simulink model "OL_HiLData"  (R2015b)
settings: Solver=FixedStepDiscrete  StartTime=0.0  StopTime=stop_time  FixedStep=step_size  RelTol=1e-3
values from neighbouring files (symbols this model uses):
  step_size = 0.1    [loadCalib.m]
  stop_time = 660    [run_test_cases.m]
undefined symbols (not defined in the file or in its folder): canChannel
libraries: canmsglib x62, canlib x29, realtime_pacer_lib x1
(part 2 of 4)

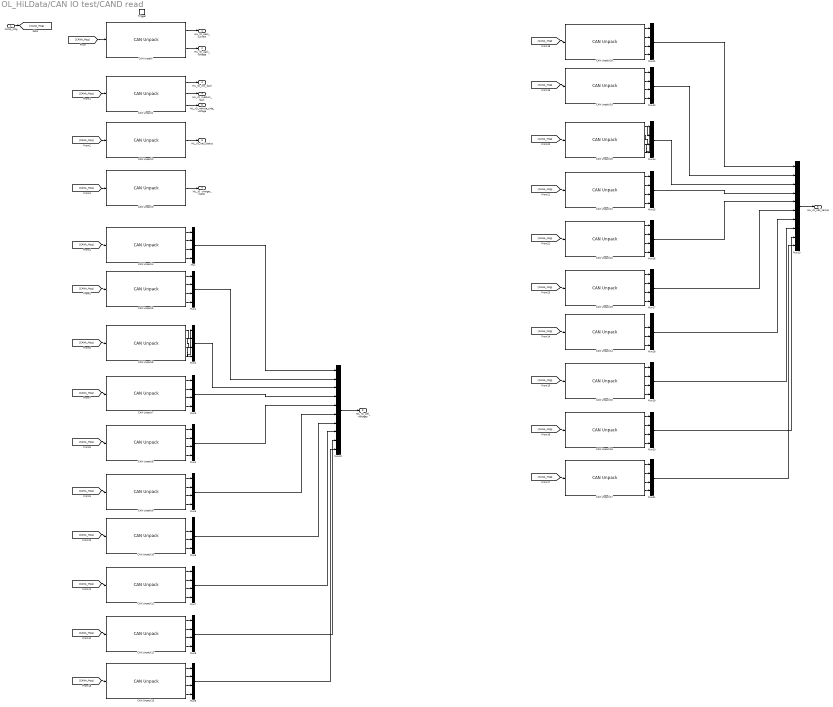
== system OL_HiLData/CAN IO test/CAND read ==
  CANA_Msg : Inport
  Trigger : TriggerPort  TriggerType=function-call  PortDimensions=1
  CAN Unpack : canmsglib/CAN Unpack  CANdbFile=D:\Projects\BMS\P006n\08_Work_in_progress\Repo_Sync_folder\HiLCANIO\IOdb.dbc  MsgList=pack_data  MsgName=pack_data  MsgIDType=Standard (11-bit identifier)  MsgIdentifier=113  MsgLength=8  SignalInfo=pack_current$16$24$2$1$1$0$1.000000e-03$0$-200$200$#pack_voltage$40$24$2$2$1$0$1.000000e-03$0$0$200$#  NSignals=2  IDPort=off  TimestampPort=off  ErrorPort=off  RemotePort=off  LengthPort=off  StatusPort=off  StartBits=str2num('[int32(16);int32(40)]')  SignalSizes=str2num('[int32(24);int32(24)]')  ByteOrders=str2num('[int32(2);int32(2)]')  DataTypes=str2num('[int32(1);int32(2)]')  MultiplexTypes=str2num('[int32(1);int32(1)]')  MultiplexValues=str2num('[double(0);double(0)]')  Factors=str2num('[double(1.000000e-03);double(1.000000e-03)]')  Offsets=str2num('[double(0);double(0)]')  Minimums=str2num('[double(-200);double(0)]')  Maximums=str2num('[double(200);double(200)]')
      settings: DataFormat=CANdb specified signals
  CAN Unpack1 : canmsglib/CAN Unpack  CANdbFile=D:\Projects\BMS\P006n\08_Work_in_progress\Repo_Sync_folder\HiLCANIO\IOdb.dbc  MsgList=pack_data_2  MsgName=pack_data_2  MsgIDType=Standard (11-bit identifier)  MsgIdentifier=114  MsgLength=8  SignalInfo=low_fault$30$1$2$2$1$0$1$0$0$1$#medium_fault$31$1$2$2$1$0$1$0$0$1$#vehicle_side_voltage$16$24$2$2$1$0$1$0$0$200$#  NSignals=3  IDPort=off  TimestampPort=off  ErrorPort=off  RemotePort=off  LengthPort=off  StatusPort=off  StartBits=str2num('[int32(30);int32(31);int32(16)]')  SignalSizes=str2num('[int32(1);int32(1);int32(24)]')  ByteOrders=str2num('[int32(2);int32(2);int32(2)]')  DataTypes=str2num('[int32(2);int32(2);int32(2)]')  MultiplexTypes=str2num('[int32(1);int32(1);int32(1)]')  MultiplexValues=str2num('[double(0);double(0);double(0)]')  Factors=str2num('[double(1);double(1);double(1)]')  Offsets=str2num('[double(0);double(0);double(0)]')  Minimums=str2num('[double(0);double(0);double(0)]')  Maximums=str2num('[double(1);double(1);double(200)]')
      settings: DataFormat=CANdb specified signals
  CAN Unpack10 : canmsglib/CAN Unpack  CANdbFile=D:\Projects\BMS\P006n\08_Work_in_progress\Repo_Sync_folder\HiLCANIO\IOdb.dbc  MsgList=cell_voltage_25_28  MsgName=cell_voltage_25_28  MsgIDType=Standard (11-bit identifier)  MsgIdentifier=86  MsgLength=8  SignalInfo=cell25_votlage$8$16$2$2$1$0$1.000000e-04$0$0$5$#cell26_votlage$24$16$2$2$1$0$1.000000e-04$0$0$5$#cell27_votlage$40$16$2$2$1$0$1.000000e-04$0$0$5$#cell28_votlage$56$16$2$2$1$0$1.000000e-04$0$0$5$#  NSignals=4  IDPort=off  TimestampPort=off  ErrorPort=off  RemotePort=off  LengthPort=off  StatusPort=off  StartBits=str2num('[int32(8);int32(24);int32(40);int32(56)]')  SignalSizes=str2num('[int32(16);int32(16);int32(16);int32(16)]')  ByteOrders=str2num('[int32(2);int32(2);int32(2);int32(2)]')  DataTypes=str2num('[int32(2);int32(2);int32(2);int32(2)]')  MultiplexTypes=str2num('[int32(1);int32(1);int32(1);int32(1)]')  MultiplexValues=str2num('[double(0);double(0);double(0);double(0)]')  Factors=str2num('[double(1.000000e-04);double(1.000000e-04);double(1.000000e-04);double(1.000000e-04)]')  Offsets=str2num('[double(0);double(0);double(0);double(0)]')  Minimums=str2num('[double(0);double(0);double(0);double(0)]')  Maximums=str2num('[double(5);double(5);double(5);double(5)]')
      settings: DataFormat=CANdb specified signals
  CAN Unpack11 : canmsglib/CAN Unpack  CANdbFile=D:\Projects\BMS\P006n\08_Work_in_progress\Repo_Sync_folder\HiLCANIO\IOdb.dbc  MsgList=cell_voltage_29_32  MsgName=cell_voltage_29_32  MsgIDType=Standard (11-bit identifier)  MsgIdentifier=87  MsgLength=8  SignalInfo=cell29_votlage$8$16$2$2$1$0$1.000000e-04$0$0$5$#cell30_votlage$24$16$2$2$1$0$1.000000e-04$0$0$5$#cell31_votlage$40$16$2$2$1$0$1.000000e-04$0$0$5$#cell32_votlage$56$16$2$2$1$0$1.000000e-04$0$0$5$#  NSignals=4  IDPort=off  TimestampPort=off  ErrorPort=off  RemotePort=off  LengthPort=off  StatusPort=off  StartBits=str2num('[int32(8);int32(24);int32(40);int32(56)]')  SignalSizes=str2num('[int32(16);int32(16);int32(16);int32(16)]')  ByteOrders=str2num('[int32(2);int32(2);int32(2);int32(2)]')  DataTypes=str2num('[int32(2);int32(2);int32(2);int32(2)]')  MultiplexTypes=str2num('[int32(1);int32(1);int32(1);int32(1)]')  MultiplexValues=str2num('[double(0);double(0);double(0);double(0)]')  Factors=str2num('[double(1.000000e-04);double(1.000000e-04);double(1.000000e-04);double(1.000000e-04)]')  Offsets=str2num('[double(0);double(0);double(0);double(0)]')  Minimums=str2num('[double(0);double(0);double(0);double(0)]')  Maximums=str2num('[double(5);double(5);double(5);double(5)]')
      settings: DataFormat=CANdb specified signals
  CAN Unpack12 : canmsglib/CAN Unpack  CANdbFile=D:\Projects\BMS\P006n\08_Work_in_progress\Repo_Sync_folder\HiLCANIO\IOdb.dbc  MsgList=cell_voltage_33_36  MsgName=cell_voltage_33_36  MsgIDType=Standard (11-bit identifier)  MsgIdentifier=88  MsgLength=8  SignalInfo=cell33_votlage$8$16$2$2$1$0$1.000000e-04$0$0$5$#cell34_votlage$24$16$2$2$1$0$1.000000e-04$0$0$5$#cell35_votlage$40$16$2$2$1$0$1.000000e-04$0$0$5$#cell36_votlage$56$16$2$2$1$0$1.000000e-04$0$0$5$#  NSignals=4  IDPort=off  TimestampPort=off  ErrorPort=off  RemotePort=off  LengthPort=off  StatusPort=off  StartBits=str2num('[int32(8);int32(24);int32(40);int32(56)]')  SignalSizes=str2num('[int32(16);int32(16);int32(16);int32(16)]')  ByteOrders=str2num('[int32(2);int32(2);int32(2);int32(2)]')  DataTypes=str2num('[int32(2);int32(2);int32(2);int32(2)]')  MultiplexTypes=str2num('[int32(1);int32(1);int32(1);int32(1)]')  MultiplexValues=str2num('[double(0);double(0);double(0);double(0)]')  Factors=str2num('[double(1.000000e-04);double(1.000000e-04);double(1.000000e-04);double(1.000000e-04)]')  Offsets=str2num('[double(0);double(0);double(0);double(0)]')  Minimums=str2num('[double(0);double(0);double(0);double(0)]')  Maximums=str2num('[double(5);double(5);double(5);double(5)]')
      settings: DataFormat=CANdb specified signals
  CAN Unpack13 : canmsglib/CAN Unpack  CANdbFile=D:\Projects\BMS\P006n\08_Work_in_progress\Repo_Sync_folder\HiLCANIO\IOdb.dbc  MsgList=cell_voltage_37_40  MsgName=cell_voltage_37_40  MsgIDType=Standard (11-bit identifier)  MsgIdentifier=89  MsgLength=8  SignalInfo=cell37_votlage$8$16$2$2$1$0$1.000000e-04$0$0$5$#cell38_votlage$24$16$2$2$1$0$1.000000e-04$0$0$5$#cell39_votlage$40$16$2$2$1$0$1.000000e-04$0$0$5$#cell40_votlage$56$16$2$2$1$0$1.000000e-04$0$0$5$#  NSignals=4  IDPort=off  TimestampPort=off  ErrorPort=off  RemotePort=off  LengthPort=off  StatusPort=off  StartBits=str2num('[int32(8);int32(24);int32(40);int32(56)]')  SignalSizes=str2num('[int32(16);int32(16);int32(16);int32(16)]')  ByteOrders=str2num('[int32(2);int32(2);int32(2);int32(2)]')  DataTypes=str2num('[int32(2);int32(2);int32(2);int32(2)]')  MultiplexTypes=str2num('[int32(1);int32(1);int32(1);int32(1)]')  MultiplexValues=str2num('[double(0);double(0);double(0);double(0)]')  Factors=str2num('[double(1.000000e-04);double(1.000000e-04);double(1.000000e-04);double(1.000000e-04)]')  Offsets=str2num('[double(0);double(0);double(0);double(0)]')  Minimums=str2num('[double(0);double(0);double(0);double(0)]')  Maximums=str2num('[double(5);double(5);double(5);double(5)]')
      settings: DataFormat=CANdb specified signals
  CAN Unpack14 : canmsglib/CAN Unpack  CANdbFile=D:\Projects\BMS\P006n\08_Work_in_progress\Repo_Sync_folder\HiLCANIO\IOdb.dbc  MsgList=cell_temp_25_28  MsgName=cell_temp_25_28  MsgIDType=Standard (11-bit identifier)  MsgIdentifier=102  MsgLength=8  SignalInfo=cell25_temperature$8$16$2$2$1$0$1.000000e-03$-20$-20$80$#cell26_temperature$24$16$2$2$1$0$1.000000e-03$-20$-20$80$#cell27_temperature$40$16$2$2$1$0$1.000000e-03$-20$-20$80$#cell28_temperature$56$16$2$2$1$0$1.000000e-03$-20$-20$80$#  NSignals=4  IDPort=off  TimestampPort=off  ErrorPort=off  RemotePort=off  LengthPort=off  StatusPort=off  StartBits=str2num('[int32(8);int32(24);int32(40);int32(56)]')  SignalSizes=str2num('[int32(16);int32(16);int32(16);int32(16)]')  ByteOrders=str2num('[int32(2);int32(2);int32(2);int32(2)]')  DataTypes=str2num('[int32(2);int32(2);int32(2);int32(2)]')  MultiplexTypes=str2num('[int32(1);int32(1);int32(1);int32(1)]')  MultiplexValues=str2num('[double(0);double(0);double(0);double(0)]')  Factors=str2num('[double(1.000000e-03);double(1.000000e-03);double(1.000000e-03);double(1.000000e-03)]')  Offsets=str2num('[double(-20);double(-20);double(-20);double(-20)]')  Minimums=str2num('[double(-20);double(-20);double(-20);double(-20)]')  Maximums=str2num('[double(80);double(80);double(80);double(80)]')
      settings: DataFormat=CANdb specified signals
  CAN Unpack15 : canmsglib/CAN Unpack  CANdbFile=D:\Projects\BMS\P006n\08_Work_in_progress\Repo_Sync_folder\HiLCANIO\IOdb.dbc  MsgList=cell_temp_29_32  MsgName=cell_temp_29_32  MsgIDType=Standard (11-bit identifier)  MsgIdentifier=103  MsgLength=8  SignalInfo=cell29_temperature$8$16$2$2$1$0$1.000000e-03$-20$-20$80$#cell30_temperature$24$16$2$2$1$0$1.000000e-03$-20$-20$80$#cell31_temperature$40$16$2$2$1$0$1.000000e-03$-20$-20$80$#cell32_temperature$56$16$2$2$1$0$1.000000e-03$-20$-20$80$#  NSignals=4  IDPort=off  TimestampPort=off  ErrorPort=off  RemotePort=off  LengthPort=off  StatusPort=off  StartBits=str2num('[int32(8);int32(24);int32(40);int32(56)]')  SignalSizes=str2num('[int32(16);int32(16);int32(16);int32(16)]')  ByteOrders=str2num('[int32(2);int32(2);int32(2);int32(2)]')  DataTypes=str2num('[int32(2);int32(2);int32(2);int32(2)]')  MultiplexTypes=str2num('[int32(1);int32(1);int32(1);int32(1)]')  MultiplexValues=str2num('[double(0);double(0);double(0);double(0)]')  Factors=str2num('[double(1.000000e-03);double(1.000000e-03);double(1.000000e-03);double(1.000000e-03)]')  Offsets=str2num('[double(-20);double(-20);double(-20);double(-20)]')  Minimums=str2num('[double(-20);double(-20);double(-20);double(-20)]')  Maximums=str2num('[double(80);double(80);double(80);double(80)]')
      settings: DataFormat=CANdb specified signals
  CAN Unpack16 : canmsglib/CAN Unpack  CANdbFile=D:\Projects\BMS\P006n\08_Work_in_progress\Repo_Sync_folder\HiLCANIO\IOdb.dbc  MsgList=cell_temp_33_36  MsgName=cell_temp_33_36  MsgIDType=Standard (11-bit identifier)  MsgIdentifier=104  MsgLength=8  SignalInfo=cell33_temperature$8$16$2$2$1$0$1.000000e-03$-20$-20$80$#cell34_temperature$24$16$2$2$1$0$1.000000e-03$-20$-20$80$#cell35_temperature$40$16$2$2$1$0$1.000000e-03$-20$-20$80$#cell36_temperature$56$16$2$2$1$0$1.000000e-03$-20$-20$80$#  NSignals=4  IDPort=off  TimestampPort=off  ErrorPort=off  RemotePort=off  LengthPort=off  StatusPort=off  StartBits=str2num('[int32(8);int32(24);int32(40);int32(56)]')  SignalSizes=str2num('[int32(16);int32(16);int32(16);int32(16)]')  ByteOrders=str2num('[int32(2);int32(2);int32(2);int32(2)]')  DataTypes=str2num('[int32(2);int32(2);int32(2);int32(2)]')  MultiplexTypes=str2num('[int32(1);int32(1);int32(1);int32(1)]')  MultiplexValues=str2num('[double(0);double(0);double(0);double(0)]')  Factors=str2num('[double(1.000000e-03);double(1.000000e-03);double(1.000000e-03);double(1.000000e-03)]')  Offsets=str2num('[double(-20);double(-20);double(-20);double(-20)]')  Minimums=str2num('[double(-20);double(-20);double(-20);double(-20)]')  Maximums=str2num('[double(80);double(80);double(80);double(80)]')
      settings: DataFormat=CANdb specified signals
  CAN Unpack17 : canmsglib/CAN Unpack  CANdbFile=D:\Projects\BMS\P006n\08_Work_in_progress\Repo_Sync_folder\HiLCANIO\IOdb.dbc  MsgList=cell_temp_37_40  MsgName=cell_temp_37_40  MsgIDType=Standard (11-bit identifier)  MsgIdentifier=105  MsgLength=8  SignalInfo=cell37_temperature$8$16$2$2$1$0$1.000000e-03$-20$-20$80$#cell38_temperature$24$16$2$2$1$0$1.000000e-03$-20$-20$80$#cell39_temperature$40$16$2$2$1$0$1.000000e-03$-20$-20$80$#cell40_temperature$56$16$2$2$1$0$1.000000e-03$-20$-20$80$#  NSignals=4  IDPort=off  TimestampPort=off  ErrorPort=off  RemotePort=off  LengthPort=off  StatusPort=off  StartBits=str2num('[int32(8);int32(24);int32(40);int32(56)]')  SignalSizes=str2num('[int32(16);int32(16);int32(16);int32(16)]')  ByteOrders=str2num('[int32(2);int32(2);int32(2);int32(2)]')  DataTypes=str2num('[int32(2);int32(2);int32(2);int32(2)]')  MultiplexTypes=str2num('[int32(1);int32(1);int32(1);int32(1)]')  MultiplexValues=str2num('[double(0);double(0);double(0);double(0)]')  Factors=str2num('[double(1.000000e-03);double(1.000000e-03);double(1.000000e-03);double(1.000000e-03)]')  Offsets=str2num('[double(-20);double(-20);double(-20);double(-20)]')  Minimums=str2num('[double(-20);double(-20);double(-20);double(-20)]')  Maximums=str2num('[double(80);double(80);double(80);double(80)]')
      settings: DataFormat=CANdb specified signals
  CAN Unpack18 : canmsglib/CAN Unpack  CANdbFile=D:\Projects\BMS\P006n\08_Work_in_progress\Repo_Sync_folder\HiLCANIO\IOdb.dbc  MsgList=cell_temp_1_4  MsgName=cell_temp_1_4  MsgIDType=Standard (11-bit identifier)  MsgIdentifier=96  MsgLength=8  SignalInfo=cell1_temperature$8$16$2$2$1$0$1.000000e-03$-20$-20$80$#cell2_temperature$24$16$2$2$1$0$1.000000e-03$-20$-20$80$#cell3_temperature$40$16$2$2$1$0$1.000000e-03$-20$-20$80$#cell4_temperature$56$16$2$2$1$0$1.000000e-03$-20$-20$80$#  NSignals=4  IDPort=off  TimestampPort=off  ErrorPort=off  RemotePort=off  LengthPort=off  StatusPort=off  StartBits=str2num('[int32(8);int32(24);int32(40);int32(56)]')  SignalSizes=str2num('[int32(16);int32(16);int32(16);int32(16)]')  ByteOrders=str2num('[int32(2);int32(2);int32(2);int32(2)]')  DataTypes=str2num('[int32(2);int32(2);int32(2);int32(2)]')  MultiplexTypes=str2num('[int32(1);int32(1);int32(1);int32(1)]')  MultiplexValues=str2num('[double(0);double(0);double(0);double(0)]')  Factors=str2num('[double(1.000000e-03);double(1.000000e-03);double(1.000000e-03);double(1.000000e-03)]')  Offsets=str2num('[double(-20);double(-20);double(-20);double(-20)]')  Minimums=str2num('[double(-20);double(-20);double(-20);double(-20)]')  Maximums=str2num('[double(80);double(80);double(80);double(80)]')
      settings: DataFormat=CANdb specified signals
  CAN Unpack19 : canmsglib/CAN Unpack  CANdbFile=D:\Projects\BMS\P006n\08_Work_in_progress\Repo_Sync_folder\HiLCANIO\IOdb.dbc  MsgList=cell_temp_5_8  MsgName=cell_temp_5_8  MsgIDType=Standard (11-bit identifier)  MsgIdentifier=97  MsgLength=8  SignalInfo=cell5_temperature$8$16$2$2$1$0$1.000000e-03$-20$-20$80$#cell6_temperature$24$16$2$2$1$0$1.000000e-03$-20$-20$80$#cell7_temperature$40$16$2$2$1$0$1.000000e-03$-20$-20$80$#cell8_temperature$56$16$2$2$1$0$1.000000e-03$-20$-20$80$#  NSignals=4  IDPort=off  TimestampPort=off  ErrorPort=off  RemotePort=off  LengthPort=off  StatusPort=off  StartBits=str2num('[int32(8);int32(24);int32(40);int32(56)]')  SignalSizes=str2num('[int32(16);int32(16);int32(16);int32(16)]')  ByteOrders=str2num('[int32(2);int32(2);int32(2);int32(2)]')  DataTypes=str2num('[int32(2);int32(2);int32(2);int32(2)]')  MultiplexTypes=str2num('[int32(1);int32(1);int32(1);int32(1)]')  MultiplexValues=str2num('[double(0);double(0);double(0);double(0)]')  Factors=str2num('[double(1.000000e-03);double(1.000000e-03);double(1.000000e-03);double(1.000000e-03)]')  Offsets=str2num('[double(-20);double(-20);double(-20);double(-20)]')  Minimums=str2num('[double(-20);double(-20);double(-20);double(-20)]')  Maximums=str2num('[double(80);double(80);double(80);double(80)]')
      settings: DataFormat=CANdb specified signals
  CAN Unpack2 : canmsglib/CAN Unpack  CANdbFile=D:\Projects\BMS\P006n\08_Work_in_progress\Repo_Sync_folder\HiLCANIO\IOdb.dbc  MsgList=driver_info  MsgName=driver_info  MsgIDType=Standard (11-bit identifier)  MsgIdentifier=115  MsgLength=8  SignalInfo=key_status$7$1$2$2$1$0$1$0$0$1$#  NSignals=1  IDPort=off  TimestampPort=off  ErrorPort=off  RemotePort=off  LengthPort=off  StatusPort=off  StartBits=str2num('[int32(7)]')  SignalSizes=str2num('[int32(1)]')  ByteOrders=str2num('[int32(2)]')  DataTypes=str2num('[int32(2)]')  MultiplexTypes=str2num('[int32(1)]')  MultiplexValues=str2num('[double(0)]')  Factors=str2num('[double(1)]')  Offsets=str2num('[double(0)]')  Minimums=str2num('[double(0)]')  Maximums=str2num('[double(1)]')
      settings: DataFormat=CANdb specified signals
  CAN Unpack20 : canmsglib/CAN Unpack  CANdbFile=D:\Projects\BMS\P006n\08_Work_in_progress\Repo_Sync_folder\HiLCANIO\IOdb.dbc  MsgList=cell_temp_9_12  MsgName=cell_temp_9_12  MsgIDType=Standard (11-bit identifier)  MsgIdentifier=98  MsgLength=8  SignalInfo=cell10_temperature$24$16$2$2$1$0$1.000000e-03$-20$-20$80$#cell11_temperature$40$16$2$2$1$0$1.000000e-03$-20$-20$80$#cell12_temperature$56$16$2$2$1$0$1.000000e-03$-20$-20$80$#cell9_temperature$8$16$2$2$1$0$1.000000e-03$-20$-20$80$#  NSignals=4  IDPort=off  TimestampPort=off  ErrorPort=off  RemotePort=off  LengthPort=off  StatusPort=off  StartBits=str2num('[int32(24);int32(40);int32(56);int32(8)]')  SignalSizes=str2num('[int32(16);int32(16);int32(16);int32(16)]')  ByteOrders=str2num('[int32(2);int32(2);int32(2);int32(2)]')  DataTypes=str2num('[int32(2);int32(2);int32(2);int32(2)]')  MultiplexTypes=str2num('[int32(1);int32(1);int32(1);int32(1)]')  MultiplexValues=str2num('[double(0);double(0);double(0);double(0)]')  Factors=str2num('[double(1.000000e-03);double(1.000000e-03);double(1.000000e-03);double(1.000000e-03)]')  Offsets=str2num('[double(-20);double(-20);double(-20);double(-20)]')  Minimums=str2num('[double(-20);double(-20);double(-20);double(-20)]')  Maximums=str2num('[double(80);double(80);double(80);double(80)]')
      settings: DataFormat=CANdb specified signals
  CAN Unpack21 : canmsglib/CAN Unpack  CANdbFile=D:\Projects\BMS\P006n\08_Work_in_progress\Repo_Sync_folder\HiLCANIO\IOdb.dbc  MsgList=cell_temp_13_16  MsgName=cell_temp_13_16  MsgIDType=Standard (11-bit identifier)  MsgIdentifier=99  MsgLength=8  SignalInfo=cell13_temperature$8$16$2$2$1$0$1.000000e-03$-20$-20$80$#cell14_temperature$24$16$2$2$1$0$1.000000e-03$-20$-20$80$#cell15_temperature$40$16$2$2$1$0$1.000000e-03$-20$-20$80$#cell16_temperature$56$16$2$2$1$0$1.000000e-03$-20$-20$80$#  NSignals=4  IDPort=off  TimestampPort=off  ErrorPort=off  RemotePort=off  LengthPort=off  StatusPort=off  StartBits=str2num('[int32(8);int32(24);int32(40);int32(56)]')  SignalSizes=str2num('[int32(16);int32(16);int32(16);int32(16)]')  ByteOrders=str2num('[int32(2);int32(2);int32(2);int32(2)]')  DataTypes=str2num('[int32(2);int32(2);int32(2);int32(2)]')  MultiplexTypes=str2num('[int32(1);int32(1);int32(1);int32(1)]')  MultiplexValues=str2num('[double(0);double(0);double(0);double(0)]')  Factors=str2num('[double(1.000000e-03);double(1.000000e-03);double(1.000000e-03);double(1.000000e-03)]')  Offsets=str2num('[double(-20);double(-20);double(-20);double(-20)]')  Minimums=str2num('[double(-20);double(-20);double(-20);double(-20)]')  Maximums=str2num('[double(80);double(80);double(80);double(80)]')
      settings: DataFormat=CANdb specified signals
  CAN Unpack22 : canmsglib/CAN Unpack  CANdbFile=D:\Projects\BMS\P006n\08_Work_in_progress\Repo_Sync_folder\HiLCANIO\IOdb.dbc  MsgList=cell_temp_17_20  MsgName=cell_temp_17_20  MsgIDType=Standard (11-bit identifier)  MsgIdentifier=100  MsgLength=8  SignalInfo=cell17_temperature$8$16$2$2$1$0$1.000000e-03$-20$-20$80$#cell18_temperature$24$16$2$2$1$0$1.000000e-03$-20$-20$80$#cell19_temperature$40$16$2$2$1$0$1.000000e-03$-20$-20$80$#cell20_temperature$56$16$2$2$1$0$1.000000e-03$-20$-20$80$#  NSignals=4  IDPort=off  TimestampPort=off  ErrorPort=off  RemotePort=off  LengthPort=off  StatusPort=off  StartBits=str2num('[int32(8);int32(24);int32(40);int32(56)]')  SignalSizes=str2num('[int32(16);int32(16);int32(16);int32(16)]')  ByteOrders=str2num('[int32(2);int32(2);int32(2);int32(2)]')  DataTypes=str2num('[int32(2);int32(2);int32(2);int32(2)]')  MultiplexTypes=str2num('[int32(1);int32(1);int32(1);int32(1)]')  MultiplexValues=str2num('[double(0);double(0);double(0);double(0)]')  Factors=str2num('[double(1.000000e-03);double(1.000000e-03);double(1.000000e-03);double(1.000000e-03)]')  Offsets=str2num('[double(-20);double(-20);double(-20);double(-20)]')  Minimums=str2num('[double(-20);double(-20);double(-20);double(-20)]')  Maximums=str2num('[double(80);double(80);double(80);double(80)]')
      settings: DataFormat=CANdb specified signals
  CAN Unpack23 : canmsglib/CAN Unpack  CANdbFile=D:\Projects\BMS\P006n\08_Work_in_progress\Repo_Sync_folder\HiLCANIO\IOdb.dbc  MsgList=cell_temp_21_24  MsgName=cell_temp_21_24  MsgIDType=Standard (11-bit identifier)  MsgIdentifier=101  MsgLength=8  SignalInfo=cell21_temperature$8$16$2$2$1$0$1.000000e-03$-20$-20$80$#cell22_temperature$24$16$2$2$1$0$1.000000e-03$-20$-20$80$#cell23_temperature$40$16$2$2$1$0$1.000000e-03$-20$-20$80$#cell24_temperature$56$16$2$2$1$0$1.000000e-03$-20$-20$80$#  NSignals=4  IDPort=off  TimestampPort=off  ErrorPort=off  RemotePort=off  LengthPort=off  StatusPort=off  StartBits=str2num('[int32(8);int32(24);int32(40);int32(56)]')  SignalSizes=str2num('[int32(16);int32(16);int32(16);int32(16)]')  ByteOrders=str2num('[int32(2);int32(2);int32(2);int32(2)]')  DataTypes=str2num('[int32(2);int32(2);int32(2);int32(2)]')  MultiplexTypes=str2num('[int32(1);int32(1);int32(1);int32(1)]')  MultiplexValues=str2num('[double(0);double(0);double(0);double(0)]')  Factors=str2num('[double(1.000000e-03);double(1.000000e-03);double(1.000000e-03);double(1.000000e-03)]')  Offsets=str2num('[double(-20);double(-20);double(-20);double(-20)]')  Minimums=str2num('[double(-20);double(-20);double(-20);double(-20)]')  Maximums=str2num('[double(80);double(80);double(80);double(80)]')
      settings: DataFormat=CANdb specified signals
  CAN Unpack3 : canmsglib/CAN Unpack  CANdbFile=D:\Projects\BMS\P006n\08_Work_in_progress\Repo_Sync_folder\HiLCANIO\IOdb.dbc  MsgList=socket_charging  MsgName=socket_charging  MsgIDType=Standard (11-bit identifier)  MsgIdentifier=112  MsgLength=8  SignalInfo=charger_signal$7$1$2$2$1$0$1$0$0$1$#  NSignals=1  IDPort=off  TimestampPort=off  ErrorPort=off  RemotePort=off  LengthPort=off  StatusPort=off  StartBits=str2num('[int32(7)]')  SignalSizes=str2num('[int32(1)]')  ByteOrders=str2num('[int32(2)]')  DataTypes=str2num('[int32(2)]')  MultiplexTypes=str2num('[int32(1)]')  MultiplexValues=str2num('[double(0)]')  Factors=str2num('[double(1)]')  Offsets=str2num('[double(0)]')  Minimums=str2num('[double(0)]')  Maximums=str2num('[double(1)]')
      settings: DataFormat=CANdb specified signals
  CAN Unpack4 : canmsglib/CAN Unpack  CANdbFile=D:\Projects\BMS\P006n\08_Work_in_progress\Repo_Sync_folder\HiLCANIO\IOdb.dbc  MsgList=cell_voltage_1_4  MsgName=cell_voltage_1_4  MsgIDType=Standard (11-bit identifier)  MsgIdentifier=80  MsgLength=8  SignalInfo=cell1_voltage$8$16$2$2$1$0$1.000000e-04$0$0$5$#cell2_voltage$24$16$2$2$1$0$1.000000e-04$0$0$5$#cell3_voltage$40$16$2$2$1$0$1.000000e-04$0$0$5$#cell4_voltage$56$16$2$2$1$0$1.000000e-04$0$0$5$#  NSignals=4  IDPort=off  TimestampPort=off  ErrorPort=off  RemotePort=off  LengthPort=off  StatusPort=off  StartBits=str2num('[int32(8);int32(24);int32(40);int32(56)]')  SignalSizes=str2num('[int32(16);int32(16);int32(16);int32(16)]')  ByteOrders=str2num('[int32(2);int32(2);int32(2);int32(2)]')  DataTypes=str2num('[int32(2);int32(2);int32(2);int32(2)]')  MultiplexTypes=str2num('[int32(1);int32(1);int32(1);int32(1)]')  MultiplexValues=str2num('[double(0);double(0);double(0);double(0)]')  Factors=str2num('[double(1.000000e-04);double(1.000000e-04);double(1.000000e-04);double(1.000000e-04)]')  Offsets=str2num('[double(0);double(0);double(0);double(0)]')  Minimums=str2num('[double(0);double(0);double(0);double(0)]')  Maximums=str2num('[double(5);double(5);double(5);double(5)]')
      settings: DataFormat=CANdb specified signals
  CAN Unpack5 : canmsglib/CAN Unpack  CANdbFile=D:\Projects\BMS\P006n\08_Work_in_progress\Repo_Sync_folder\HiLCANIO\IOdb.dbc  MsgList=cell_voltage_5_8  MsgName=cell_voltage_5_8  MsgIDType=Standard (11-bit identifier)  MsgIdentifier=81  MsgLength=8  SignalInfo=cell5_votlage$8$16$2$2$1$0$1.000000e-04$0$0$5$#cell6_voltage$24$16$2$2$1$0$1.000000e-04$0$0$5$#cell7_voltage$40$16$2$2$1$0$1.000000e-04$0$0$5$#cell8_voltage$56$16$2$2$1$0$1.000000e-04$0$0$5$#  NSignals=4  IDPort=off  TimestampPort=off  ErrorPort=off  RemotePort=off  LengthPort=off  StatusPort=off  StartBits=str2num('[int32(8);int32(24);int32(40);int32(56)]')  SignalSizes=str2num('[int32(16);int32(16);int32(16);int32(16)]')  ByteOrders=str2num('[int32(2);int32(2);int32(2);int32(2)]')  DataTypes=str2num('[int32(2);int32(2);int32(2);int32(2)]')  MultiplexTypes=str2num('[int32(1);int32(1);int32(1);int32(1)]')  MultiplexValues=str2num('[double(0);double(0);double(0);double(0)]')  Factors=str2num('[double(1.000000e-04);double(1.000000e-04);double(1.000000e-04);double(1.000000e-04)]')  Offsets=str2num('[double(0);double(0);double(0);double(0)]')  Minimums=str2num('[double(0);double(0);double(0);double(0)]')  Maximums=str2num('[double(5);double(5);double(5);double(5)]')
      settings: DataFormat=CANdb specified signals
  CAN Unpack6 : canmsglib/CAN Unpack  CANdbFile=D:\Projects\BMS\P006n\08_Work_in_progress\Repo_Sync_folder\HiLCANIO\IOdb.dbc  MsgList=cell_voltage_9_12  MsgName=cell_voltage_9_12  MsgIDType=Standard (11-bit identifier)  MsgIdentifier=82  MsgLength=8  SignalInfo=cell10_voltage$24$16$2$2$1$0$1.000000e-04$0$0$5$#cell11_voltage$40$16$2$2$1$0$1.000000e-04$0$0$5$#cell12_voltage$56$16$2$2$1$0$1.000000e-04$0$0$5$#cell9_votlage$8$16$2$2$1$0$1.000000e-04$0$0$5$#  NSignals=4  IDPort=off  TimestampPort=off  ErrorPort=off  RemotePort=off  LengthPort=off  StatusPort=off  StartBits=str2num('[int32(24);int32(40);int32(56);int32(8)]')  SignalSizes=str2num('[int32(16);int32(16);int32(16);int32(16)]')  ByteOrders=str2num('[int32(2);int32(2);int32(2);int32(2)]')  DataTypes=str2num('[int32(2);int32(2);int32(2);int32(2)]')  MultiplexTypes=str2num('[int32(1);int32(1);int32(1);int32(1)]')  MultiplexValues=str2num('[double(0);double(0);double(0);double(0)]')  Factors=str2num('[double(1.000000e-04);double(1.000000e-04);double(1.000000e-04);double(1.000000e-04)]')  Offsets=str2num('[double(0);double(0);double(0);double(0)]')  Minimums=str2num('[double(0);double(0);double(0);double(0)]')  Maximums=str2num('[double(5);double(5);double(5);double(5)]')
      settings: DataFormat=CANdb specified signals
  CAN Unpack7 : canmsglib/CAN Unpack  CANdbFile=D:\Projects\BMS\P006n\08_Work_in_progress\Repo_Sync_folder\HiLCANIO\IOdb.dbc  MsgList=cell_voltage_13_16  MsgName=cell_voltage_13_16  MsgIDType=Standard (11-bit identifier)  MsgIdentifier=83  MsgLength=8  SignalInfo=cell13_votlage$8$16$2$2$1$0$1.000000e-04$0$0$5$#cell14_voltage$24$16$2$2$1$0$1.000000e-04$0$0$5$#cell15_voltage$40$16$2$2$1$0$1.000000e-04$0$0$5$#cell16_voltage$56$16$2$2$1$0$1.000000e-04$0$0$5$#  NSignals=4  IDPort=off  TimestampPort=off  ErrorPort=off  RemotePort=off  LengthPort=off  StatusPort=off  StartBits=str2num('[int32(8);int32(24);int32(40);int32(56)]')  SignalSizes=str2num('[int32(16);int32(16);int32(16);int32(16)]')  ByteOrders=str2num('[int32(2);int32(2);int32(2);int32(2)]')  DataTypes=str2num('[int32(2);int32(2);int32(2);int32(2)]')  MultiplexTypes=str2num('[int32(1);int32(1);int32(1);int32(1)]')  MultiplexValues=str2num('[double(0);double(0);double(0);double(0)]')  Factors=str2num('[double(1.000000e-04);double(1.000000e-04);double(1.000000e-04);double(1.000000e-04)]')  Offsets=str2num('[double(0);double(0);double(0);double(0)]')  Minimums=str2num('[double(0);double(0);double(0);double(0)]')  Maximums=str2num('[double(5);double(5);double(5);double(5)]')
      settings: DataFormat=CANdb specified signals
  CAN Unpack8 : canmsglib/CAN Unpack  CANdbFile=D:\Projects\BMS\P006n\08_Work_in_progress\Repo_Sync_folder\HiLCANIO\IOdb.dbc  MsgList=cell_voltage_17_20  MsgName=cell_voltage_17_20  MsgIDType=Standard (11-bit identifier)  MsgIdentifier=84  MsgLength=8  SignalInfo=cell17_votlage$8$16$2$2$1$0$1.000000e-04$0$0$5$#cell18_voltage$24$16$2$2$1$0$1.000000e-04$0$0$5$#cell19_voltage$40$16$2$2$1$0$1.000000e-04$0$0$5$#cell20_voltage$56$16$2$2$1$0$1.000000e-04$0$0$5$#  NSignals=4  IDPort=off  TimestampPort=off  ErrorPort=off  RemotePort=off  LengthPort=off  StatusPort=off  StartBits=str2num('[int32(8);int32(24);int32(40);int32(56)]')  SignalSizes=str2num('[int32(16);int32(16);int32(16);int32(16)]')  ByteOrders=str2num('[int32(2);int32(2);int32(2);int32(2)]')  DataTypes=str2num('[int32(2);int32(2);int32(2);int32(2)]')  MultiplexTypes=str2num('[int32(1);int32(1);int32(1);int32(1)]')  MultiplexValues=str2num('[double(0);double(0);double(0);double(0)]')  Factors=str2num('[double(1.000000e-04);double(1.000000e-04);double(1.000000e-04);double(1.000000e-04)]')  Offsets=str2num('[double(0);double(0);double(0);double(0)]')  Minimums=str2num('[double(0);double(0);double(0);double(0)]')  Maximums=str2num('[double(5);double(5);double(5);double(5)]')
      settings: DataFormat=CANdb specified signals
  CAN Unpack9 : canmsglib/CAN Unpack  CANdbFile=D:\Projects\BMS\P006n\08_Work_in_progress\Repo_Sync_folder\HiLCANIO\IOdb.dbc  MsgList=cell_voltage_21_24  MsgName=cell_voltage_21_24  MsgIDType=Standard (11-bit identifier)  MsgIdentifier=85  MsgLength=8  SignalInfo=cell21_votlage$8$16$2$2$1$0$1.000000e-04$0$0$5$#cell22_votlage$24$16$2$2$1$0$1.000000e-04$0$0$5$#cell23_votlage$40$16$2$2$1$0$1.000000e-04$0$0$5$#cell24_votlage$56$16$2$2$1$0$1.000000e-04$0$0$5$#  NSignals=4  IDPort=off  TimestampPort=off  ErrorPort=off  RemotePort=off  LengthPort=off  StatusPort=off  StartBits=str2num('[int32(8);int32(24);int32(40);int32(56)]')  SignalSizes=str2num('[int32(16);int32(16);int32(16);int32(16)]')  ByteOrders=str2num('[int32(2);int32(2);int32(2);int32(2)]')  DataTypes=str2num('[int32(2);int32(2);int32(2);int32(2)]')  MultiplexTypes=str2num('[int32(1);int32(1);int32(1);int32(1)]')  MultiplexValues=str2num('[double(0);double(0);double(0);double(0)]')  Factors=str2num('[double(1.000000e-04);double(1.000000e-04);double(1.000000e-04);double(1.000000e-04)]')  Offsets=str2num('[double(0);double(0);double(0);double(0)]')  Minimums=str2num('[double(0);double(0);double(0);double(0)]')  Maximums=str2num('[double(5);double(5);double(5);double(5)]')
      settings: DataFormat=CANdb specified signals
  Mux{,1..9,11..12,14..21} (20 alike) : Mux
  Mux10 : Mux  Inputs=10
  Mux13 : Mux  Inputs=10
  HIL_IO_pack_current : Outport
  HIL_IO_pack_voltage : Outport  Port=2
  HIL_IO_low_fault : Outport  Port=3
  HIL_IO_medium_fault : Outport  Port=4
  HIL_IO_vehicle_side_voltage : Outport  Port=5
  HIL_IO_key_status : Outport  Port=6
  HIL_IO_charger_signal : Outport  Port=7
  HIL_IO_cell_voltages : Outport  Port=8
  HIL_IO_cell_temps : Outport  Port=9
  wires:
  CANA_Msg/1 -> [CANA_Msg]
  [CANA_Msg] -> CAN Unpack/1
  [CANA_Msg] -> CAN Unpack1/1
  [CANA_Msg] -> CAN Unpack2/1
  [CANA_Msg] -> CAN Unpack3/1
  [CANA_Msg] -> CAN Unpack4/1
  [CANA_Msg] -> CAN Unpack5/1
  [CANA_Msg] -> CAN Unpack6/1
  [CANA_Msg] -> CAN Unpack7/1
  [CANA_Msg] -> CAN Unpack8/1
  [CANA_Msg] -> CAN Unpack9/1
  [CANA_Msg] -> CAN Unpack10/1
  [CANA_Msg] -> CAN Unpack11/1
  [CANA_Msg] -> CAN Unpack12/1
  [CANA_Msg] -> CAN Unpack13/1
  CAN Unpack4/1 -> Mux/1
  CAN Unpack4/2 -> Mux/2
  CAN Unpack4/3 -> Mux/3
  CAN Unpack4/4 -> Mux/4
  CAN Unpack5/1 -> Mux1/1
  CAN Unpack5/2 -> Mux1/2
  CAN Unpack5/3 -> Mux1/3
  CAN Unpack5/4 -> Mux1/4
  CAN Unpack7/1 -> Mux3/1
  CAN Unpack7/2 -> Mux3/2
  CAN Unpack7/3 -> Mux3/3
  CAN Unpack7/4 -> Mux3/4
  CAN Unpack8/1 -> Mux4/1
  CAN Unpack8/2 -> Mux4/2
  CAN Unpack8/3 -> Mux4/3
  CAN Unpack8/4 -> Mux4/4
  CAN Unpack9/1 -> Mux5/1
  CAN Unpack9/2 -> Mux5/2
  CAN Unpack9/3 -> Mux5/3
  CAN Unpack9/4 -> Mux5/4
  CAN Unpack10/2 -> Mux6/2
  CAN Unpack10/3 -> Mux6/3
  CAN Unpack10/4 -> Mux6/4
  CAN Unpack11/1 -> Mux7/1
  CAN Unpack11/2 -> Mux7/2
  CAN Unpack11/3 -> Mux7/3
  CAN Unpack11/4 -> Mux7/4
  CAN Unpack12/1 -> Mux8/1
  CAN Unpack12/2 -> Mux8/2
  CAN Unpack12/3 -> Mux8/3
  CAN Unpack12/4 -> Mux8/4
  CAN Unpack13/1 -> Mux9/1
  CAN Unpack13/2 -> Mux9/2
  CAN Unpack13/3 -> Mux9/3
  CAN Unpack13/4 -> Mux9/4
  CAN Unpack6/4 -> Mux2/1
  CAN Unpack6/1 -> Mux2/2
  CAN Unpack6/2 -> Mux2/3
  CAN Unpack6/3 -> Mux2/4
  Mux/1 -> Mux10/1
  Mux1/1 -> Mux10/2
  Mux2/1 -> Mux10/3
  Mux3/1 -> Mux10/4
  Mux4/1 -> Mux10/5
  Mux5/1 -> Mux10/6
  Mux6/1 -> Mux10/7
  Mux7/1 -> Mux10/8
  Mux8/1 -> Mux10/9
  Mux9/1 -> Mux10/10
  [CANA_Msg] -> CAN Unpack18/1
  [CANA_Msg] -> CAN Unpack19/1
  [CANA_Msg] -> CAN Unpack20/1
  [CANA_Msg] -> CAN Unpack21/1
  [CANA_Msg] -> CAN Unpack22/1
  [CANA_Msg] -> CAN Unpack23/1
  [CANA_Msg] -> CAN Unpack14/1
  [CANA_Msg] -> CAN Unpack15/1
  [CANA_Msg] -> CAN Unpack16/1
  [CANA_Msg] -> CAN Unpack17/1
  CAN Unpack18/1 -> Mux11/1
  CAN Unpack18/2 -> Mux11/2
  CAN Unpack18/3 -> Mux11/3
  CAN Unpack18/4 -> Mux11/4
  CAN Unpack19/1 -> Mux12/1
  CAN Unpack19/2 -> Mux12/2
  CAN Unpack19/3 -> Mux12/3
  CAN Unpack19/4 -> Mux12/4
  CAN Unpack21/1 -> Mux15/1
  CAN Unpack21/2 -> Mux15/2
  CAN Unpack21/3 -> Mux15/3
  CAN Unpack21/4 -> Mux15/4
  CAN Unpack22/1 -> Mux16/1
  CAN Unpack22/2 -> Mux16/2
  CAN Unpack22/3 -> Mux16/3
  CAN Unpack22/4 -> Mux16/4
  CAN Unpack23/1 -> Mux17/1
  CAN Unpack23/2 -> Mux17/2
  CAN Unpack23/3 -> Mux17/3
  CAN Unpack23/4 -> Mux17/4
  CAN Unpack14/2 -> Mux18/2
  CAN Unpack14/3 -> Mux18/3
  CAN Unpack14/4 -> Mux18/4
  CAN Unpack15/1 -> Mux19/1
  CAN Unpack15/2 -> Mux19/2
  CAN Unpack15/3 -> Mux19/3
  CAN Unpack15/4 -> Mux19/4
  CAN Unpack16/1 -> Mux20/1
  CAN Unpack16/2 -> Mux20/2
  CAN Unpack16/3 -> Mux20/3
  CAN Unpack16/4 -> Mux20/4
  CAN Unpack17/1 -> Mux21/1
  CAN Unpack17/2 -> Mux21/2
  CAN Unpack17/3 -> Mux21/3
  CAN Unpack17/4 -> Mux21/4
  CAN Unpack20/4 -> Mux14/1
  CAN Unpack20/1 -> Mux14/2
  CAN Unpack20/2 -> Mux14/3
  CAN Unpack20/3 -> Mux14/4
  Mux11/1 -> Mux13/1
  Mux12/1 -> Mux13/2
  Mux14/1 -> Mux13/3
  Mux15/1 -> Mux13/4
  Mux16/1 -> Mux13/5
  Mux17/1 -> Mux13/6
  Mux18/1 -> Mux13/7
  Mux19/1 -> Mux13/8
  Mux20/1 -> Mux13/9
  Mux21/1 -> Mux13/10
  CAN Unpack/1 -> HIL_IO_pack_current/1
  CAN Unpack/2 -> HIL_IO_pack_voltage/1
  CAN Unpack1/1 -> HIL_IO_low_fault/1
  CAN Unpack1/2 -> HIL_IO_medium_fault/1
  CAN Unpack1/3 -> HIL_IO_vehicle_side_voltage/1
  CAN Unpack2/1 -> HIL_IO_key_status/1
  CAN Unpack3/1 -> HIL_IO_charger_signal/1
  Mux10/1 -> HIL_IO_cell_voltages/1
  Mux13/1 -> HIL_IO_cell_temps/1
